simulink library "SEWSYS_library"  (Simulink 6.0)
settings: Solver=ode45  SolverMode=SingleTasking  StartTime=0.0  StopTime=10.0  RelTol=1e-3
values from neighbouring files (symbols this model uses):
  sec_per_ts = in_sec_per_ts    [Prep.m]
undefined symbols (not defined in the file or in its folder): DiscIntNeverNeededParam
settings Model: LastModifiedBy=v94ahlst
settings OptimizationCC: BooleanDataType=off
settings DebuggingCC: SolverPrmCheckMsg=none
settings HardwareCC: TargetUnknown=on

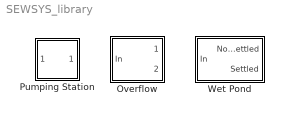
== system SEWSYS_library ==
  Overflow : Subsystem  mask(Overflow){choice=off, limit=0}
      mask prompts: choice "Overflow active"; limit "Overflow limit [m3/s]"
      mask help: Models an overflow
      mask Help:
      | To model an overflow:
      | First make the overflow active by the checkbox. Then enter the Overflow limit, ie the discharge threshold for which the overflow starts diverting. The signal from the first outport contains the bypassed part, the second outport the transit part.
  Pumping Station : Subsystem  mask(Pump){qp=, Ap=, ystart=, ynod=, ts=sec_per_ts}
      mask prompts: qp "Pump Capacity [m³/s]"; Ap "Pumping Pit Area [m²]"; ystart "Start Level [m] (Stop Level is ±0 m)"; ynod "Emergency Overflow Level [m]"; ts "Seconds per Timestep (DO NOT CHANGE THIS!)"
      mask help: Models a pumping station.
      mask Help: Enter the parameters
      mask Display: plot([0 1 5 6], [0 0 4 4])
  Wet Pond : Subsystem  mask(Wet Pond){Ap=0, d=0, n=1, vs=1.4977e-004, q_threshold=0.02, ts=sec_per_ts}
      mask prompts: Ap "Pond Area [m2]"; d "Average pond depth [m]"; n "Turbulence constant, n=1 poor performance (variable inflow)"; vs "Average settling velocity [m/s]"; q_threshold "Limit for dynamic settling [m3/s]"; ts "Seconds per Timestep (DO NOT CHANGE THIS!)"
      mask init:
      | partboundSS=[ ;% uncertain values, calculated from measurements (Pettersson et al, 1999 p.870)
      |    0.57      ;% P-tot
      |    0.10      ;% Tot-N
      |    0         ;% NH3/NH4-N
      |    0         ;% NO3-N
      |    0         ;% N2O-N
      |    0         ;% SS
      |    0.57      ;% BOD
      |    0         ;% COD
      |    0         ;% C-tot
      |    0         ;% Phase index
      |    0.43      ;% Cu
      |    0.43      ;% Zn
      |    0.71      ;% Pb
      |    0.16      ;% Cd
      |    0         ;% Hg
      |    0         ;% Cr
      |    0.90	    ;% Pt assumed values
      |    0.90	    ;% Pd ---"---
      |    0.90		 ;% Rh ---"---
      |    0.85      ;% PAH
      |    ]';

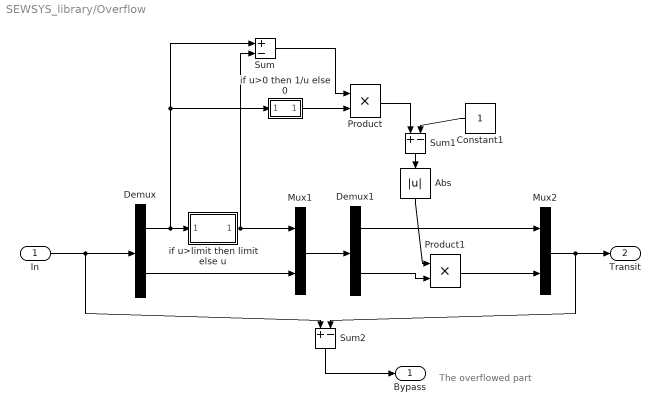
== system SEWSYS_library/Overflow ==
  note: The overflowed part
  In : Inport  Port=1  LatchInput=off
  Abs : Abs  Orientation=down  SaturateOnIntegerOverflow=on
  Constant1 : Constant  Orientation=left
  Demux : Demux  Outputs=[1 -1]
  Demux1 : Demux  Outputs=[1 -1]
  Mux1 : Mux  Inputs=2
  Mux2 : Mux  Inputs=2
  Product : Product  SaturateOnIntegerOverflow=on  InputSameDT=on
  Product1 : Product  SaturateOnIntegerOverflow=on  InputSameDT=on
  Sum : Sum  Inputs=+-  SaturateOnIntegerOverflow=on  InputSameDT=on
  Sum1 : Sum  Orientation=down  Inputs=+-  SaturateOnIntegerOverflow=on  InputSameDT=on
  Sum2 : Sum  Orientation=down  Inputs=+-  SaturateOnIntegerOverflow=on  InputSameDT=on
  if u>0 then 1/u else 0 : Subsystem
      mask Display: disp('1/u')
  if u>limit then limit else u : Subsystem
      mask Display: disp('Overflow')
  Bypass : Outport
  Transit : Outport  Port=2
  wires:
  Demux/2 -> Mux1/2
  Mux1/1 -> Demux1/1
  Demux1/1 -> Mux2/1
  Demux1/2 -> Product1/2
  Product1/1 -> Mux2/2
  if u>limit then limit else u/1(out_1) -> Sum/2, Mux1/1
  Constant1/1 -> Sum1/2
  Demux/1 -> if u>limit then limit else u/1(in_1), Sum/1, if u>0 then 1/u else 0/1(in_1)
  Sum1/1 -> Abs/1
  if u>0 then 1/u else 0/1(out_1) -> Product/2
  Sum2/1 -> Bypass/1
  In/1 -> Demux/1, Sum2/1
  Mux2/1 -> Transit/1, Sum2/2
  Product/1 -> Sum1/1
  Abs/1 -> Product1/1
  Sum/1 -> Product/1

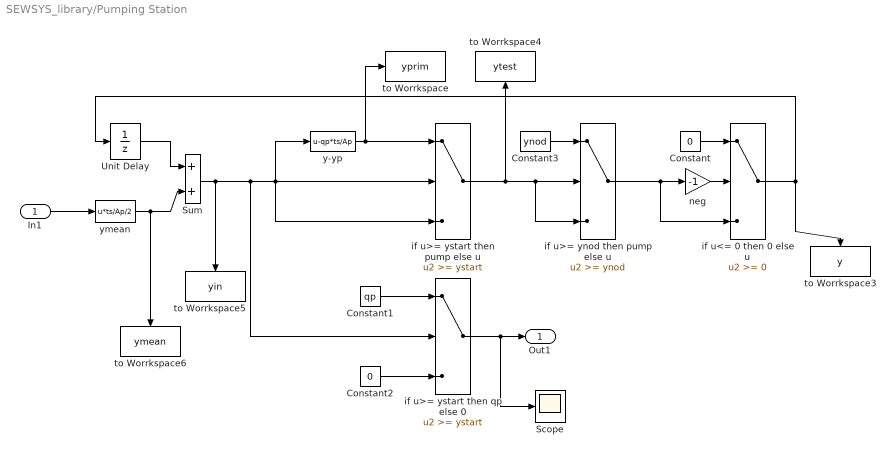
== system SEWSYS_library/Pumping Station ==
  In1 : Inport  Port=1  LatchInput=off
  Constant : Constant  Value=0
  Constant1 : Constant  Value=qp
  Constant2 : Constant  Value=0
  Constant3 : Constant  Value=ynod
  Scope : Scope
  Sum : Sum  SaturateOnIntegerOverflow=on  InputSameDT=on
  Unit Delay : UnitDelay
  if u<= 0 then 0 else u : Switch  SaturateOnIntegerOverflow=on  InputSameDT=on
  if u>= ynod then pump else u : Switch  Threshold=ynod  SaturateOnIntegerOverflow=on  InputSameDT=on
  if u>= ystart then pump else u : Switch  Threshold=ystart  SaturateOnIntegerOverflow=on  InputSameDT=on
  if u>= ystart then qp else 0 : Switch  Threshold=ystart  SaturateOnIntegerOverflow=on  InputSameDT=on
  neg : Gain  Gain=-1  SaturateOnIntegerOverflow=on
  to Worrkspace : ToWorkspace  VariableName=yprim  SampleTime=-1  SaveFormat=Array
  to Worrkspace3 : ToWorkspace  VariableName=y  SampleTime=-1  SaveFormat=Array
      settings: Orientation=down
  to Worrkspace4 : ToWorkspace  VariableName=ytest  SampleTime=-1  SaveFormat=Array
      settings: Orientation=up
  to Worrkspace5 : ToWorkspace  VariableName=yin  SampleTime=-1  SaveFormat=Array
      settings: Orientation=down
  to Worrkspace6 : ToWorkspace  VariableName=ymean  SampleTime=-1  SaveFormat=Array
      settings: Orientation=down
  y-yp : Fcn  Expr=u-qp*ts/Ap
  ymean : Fcn  Expr=u*ts/Ap/2
  Out1 : Outport
  wires:
  In1/1 -> ymean/1
  if u>= ystart then qp else 0/1 -> Scope/1, Out1/1
  Constant3/1 -> if u>= ynod then pump else u/1
  if u>= ystart then pump else u/1 -> if u>= ynod then pump else u/3, if u>= ynod then pump else u/2, to Worrkspace4/1
  if u>= ynod then pump else u/1 -> if u<= 0 then 0 else u/3, neg/1
  if u<= 0 then 0 else u/1 -> to Worrkspace3/1, Unit Delay/1
  neg/1 -> if u<= 0 then 0 else u/2
  Constant/1 -> if u<= 0 then 0 else u/1
  ymean/1 -> to Worrkspace6/1, Sum/2
  Constant2/1 -> if u>= ystart then qp else 0/3
  Constant1/1 -> if u>= ystart then qp else 0/1
  Sum/1 -> if u>= ystart then qp else 0/2, y-yp/1, if u>= ystart then pump else u/3, if u>= ystart then pump else u/2, to Worrkspace5/1
  y-yp/1 -> to Worrkspace/1, if u>= ystart then pump else u/1
  Unit Delay/1 -> Sum/1

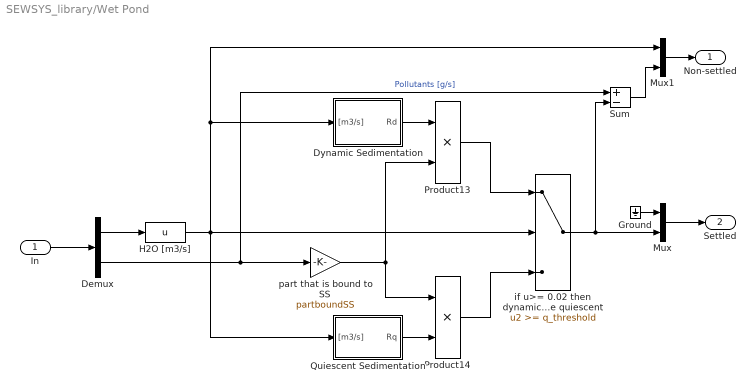
== system SEWSYS_library/Wet Pond ==
  In : Inport  Port=1  LatchInput=off
  Demux : Demux  Outputs=[1 -1]
  Dynamic Sedimentation : Subsystem
  Ground : Ground
  H2O [m3/s] : Fcn  Expr=u
  Mux : Mux  Inputs=2
  Mux1 : Mux  Inputs=2
  Product13 : Product  SaturateOnIntegerOverflow=on  InputSameDT=on
  Product14 : Product  SaturateOnIntegerOverflow=on  InputSameDT=on
  Quiescent Sedimentation : Subsystem
  Sum : Sum  Inputs=+-  SaturateOnIntegerOverflow=on  InputSameDT=on
  if u>= 0.02 then dynamic else quiescent : Switch  Threshold=q_threshold  SaturateOnIntegerOverflow=on  InputSameDT=on
  part that is bound to SS : Gain  Gain=partboundSS  SaturateOnIntegerOverflow=on
  Non-settled : Outport
  Settled : Outport  Port=2
  wires:
  part that is bound to SS/1 -> Product13/2, Product14/1
  Demux/2 -> part that is bound to SS/1, Sum/1  "Pollutants [g/s]"
  Mux1/1 -> Non-settled/1
  Sum/1 -> Mux1/2
  if u>= 0.02 then dynamic else quiescent/1 -> Sum/2, Mux/2
  Ground/1 -> Mux/1
  Mux/1 -> Settled/1
  Product14/1 -> if u>= 0.02 then dynamic else quiescent/3
  Product13/1 -> if u>= 0.02 then dynamic else quiescent/1
  Quiescent Sedimentation/1(Rq) -> Product14/2
  Dynamic Sedimentation/1(Rd) -> Product13/1
  In/1 -> Demux/1
  Demux/1 -> H2O [m3/s]/1
  H2O [m3/s]/1 -> Mux1/1, Dynamic Sedimentation/1("[m3/s]"), Quiescent Sedimentation/1("[m3/s]"), if u>= 0.02 then dynamic else quiescent/2

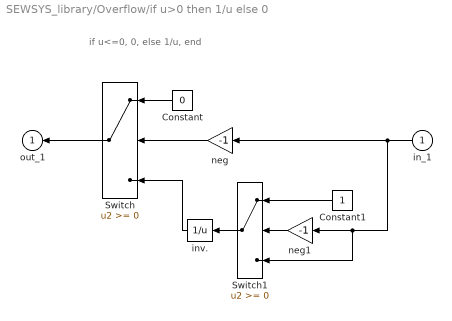
== system SEWSYS_library/Overflow/if u>0 then 1/u else 0 ==
  note: if u<=0, 0, else 1/u, end
  in_1 : Inport  Orientation=left  Port=1  LatchInput=off
  Constant : Constant  Orientation=left  Value=0
  Constant1 : Constant  Orientation=left
  Switch : Switch  Orientation=left  SaturateOnIntegerOverflow=on  InputSameDT=on
  Switch1 : Switch  Orientation=left  SaturateOnIntegerOverflow=on  InputSameDT=on
  inv. : Fcn  Orientation=left  Expr=1/u
  neg : Gain  Orientation=left  Gain=-1  SaturateOnIntegerOverflow=on
  neg1 : Gain  Orientation=left  Gain=-1  SaturateOnIntegerOverflow=on
  out_1 : Outport  Orientation=left  InitialOutput=0
  wires:
  Constant/1 -> Switch/1
  neg/1 -> Switch/2
  Switch/1 -> out_1/1
  inv./1 -> Switch/3
  Switch1/1 -> inv./1
  neg1/1 -> Switch1/2
  Constant1/1 -> Switch1/1
  in_1/1 -> neg/1, neg1/1, Switch1/3

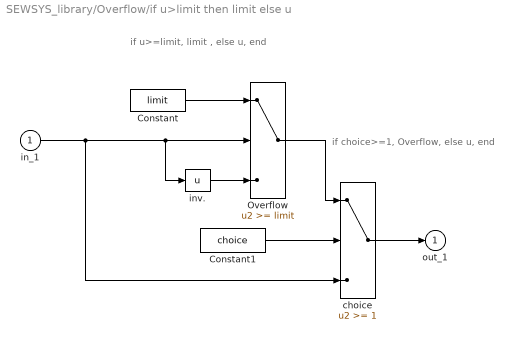
== system SEWSYS_library/Overflow/if u>limit then limit else u ==
  note: if u>=limit, limit
      | , else u, end
  note: if choice>=1, Overflow, else u, end
  in_1 : Inport  Port=1  LatchInput=off
  Constant : Constant  Value=limit
  Constant1 : Constant  Value=choice
  Overflow : Switch  Threshold=limit  SaturateOnIntegerOverflow=on  InputSameDT=on
  choice : Switch  Threshold=1  SaturateOnIntegerOverflow=on  InputSameDT=on
  inv. : Fcn  Expr=u
  out_1 : Outport  InitialOutput=0
  wires:
  Constant1/1 -> choice/2
  Constant/1 -> Overflow/1
  inv./1 -> Overflow/3
  Overflow/1 -> choice/1
  in_1/1 -> Overflow/2, inv./1, choice/3
  choice/1 -> out_1/1

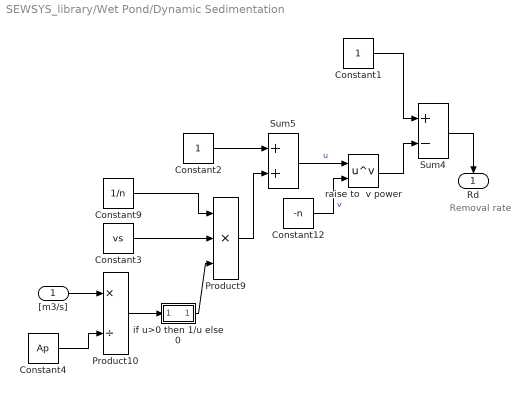
== system SEWSYS_library/Wet Pond/Dynamic Sedimentation ==
  note: Removal rate
  "[m3/s]" : Inport  Port=1  LatchInput=off
  Constant1 : Constant
  Constant12 : Constant  Value=-n
  Constant2 : Constant
  Constant3 : Constant  Value=vs
  Constant4 : Constant  Value=Ap
  Constant9 : Constant  Value=1/n
  Product10 : Product  Inputs=*/  SaturateOnIntegerOverflow=on  InputSameDT=on
  Product9 : Product  Inputs=3  SaturateOnIntegerOverflow=on  InputSameDT=on
  Sum4 : Sum  Inputs=+-  SaturateOnIntegerOverflow=on  InputSameDT=on
  Sum5 : Sum  SaturateOnIntegerOverflow=on  InputSameDT=on
  if u>0 then 1/u else 0 : Subsystem
      mask Display: disp('1/u')
  raise to  v power : Math  Operator=pow  SaturateOnIntegerOverflow=on
  Rd : Outport  Orientation=down
  wires:
  "[m3/s]"/1 -> Product10/1
  Constant4/1 -> Product10/2
  Product10/1 -> if u>0 then 1/u else 0/1(in_1)
  if u>0 then 1/u else 0/1(out_1) -> Product9/3
  Constant12/1 -> raise to  v power/2  "v"
  Constant9/1 -> Product9/1
  Constant3/1 -> Product9/2
  Product9/1 -> Sum5/2
  Constant2/1 -> Sum5/1
  Sum5/1 -> raise to  v power/1  "u"
  raise to  v power/1 -> Sum4/2
  Sum4/1 -> Rd/1
  Constant1/1 -> Sum4/1

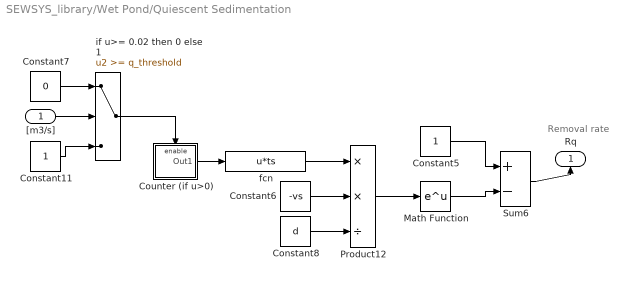
== system SEWSYS_library/Wet Pond/Quiescent Sedimentation ==
  note: Removal rate
  "[m3/s]" : Inport  Port=1  LatchInput=off
  Constant11 : Constant
  Constant5 : Constant
  Constant6 : Constant  Value=-vs
  Constant7 : Constant  Value=0
  Constant8 : Constant  Value=d
  Counter (if u>0) : Subsystem  TreatAsAtomicUnit=on
  Math Function : Math  SaturateOnIntegerOverflow=on
  Product12 : Product  Inputs=**/  SaturateOnIntegerOverflow=on  InputSameDT=on
  Sum6 : Sum  Inputs=+-  SaturateOnIntegerOverflow=on  InputSameDT=on
  fcn : Fcn  Expr=u*ts
  if u>= 0.02 then 0 else 1 : Switch  Threshold=q_threshold  SaturateOnIntegerOverflow=on  InputSameDT=on
  Rq : Outport  Orientation=up
  wires:
  Counter (if u>0)/1(Out1) -> fcn/1
  "[m3/s]"/1 -> if u>= 0.02 then 0 else 1/2
  if u>= 0.02 then 0 else 1/1 -> Counter (if u>0)/Enable
  Constant7/1 -> if u>= 0.02 then 0 else 1/1
  Constant11/1 -> if u>= 0.02 then 0 else 1/3
  fcn/1 -> Product12/1
  Constant8/1 -> Product12/3
  Constant6/1 -> Product12/2
  Product12/1 -> Math Function/1
  Constant5/1 -> Sum6/1
  Sum6/1 -> Rq/1
  Math Function/1 -> Sum6/2

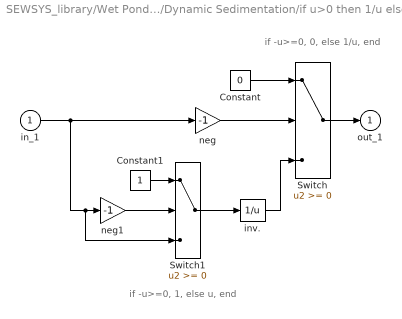
== system SEWSYS_library/Wet Pond/Dynamic Sedimentation/if u>0 then 1/u else 0 ==
  note: if -u>=0, 0, else 1/u, end
  note: if -u>=0, 1, else u, end
  in_1 : Inport  Port=1  LatchInput=off
  Constant : Constant  Value=0
  Constant1 : Constant
  Switch : Switch  SaturateOnIntegerOverflow=on  InputSameDT=on
  Switch1 : Switch  SaturateOnIntegerOverflow=on  InputSameDT=on
  inv. : Fcn  Expr=1/u
  neg : Gain  Gain=-1  SaturateOnIntegerOverflow=on
  neg1 : Gain  Gain=-1  SaturateOnIntegerOverflow=on
  out_1 : Outport  InitialOutput=0
  wires:
  Constant/1 -> Switch/1
  neg/1 -> Switch/2
  Switch/1 -> out_1/1
  inv./1 -> Switch/3
  Switch1/1 -> inv./1
  Constant1/1 -> Switch1/1
  neg1/1 -> Switch1/2
  in_1/1 -> neg/1, neg1/1, Switch1/3

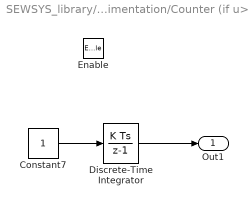
== system SEWSYS_library/Wet Pond/Quiescent Sedimentation/Counter (if u>0) ==
  Enable : EnablePort  StatesWhenEnabling=reset
  Constant7 : Constant
  Discrete-Time Integrator : DiscreteIntegrator  InitialCondition=1  ICPrevOutput=DiscIntNeverNeededParam  ICPrevScaledInput=DiscIntNeverNeededParam
  Out1 : Outport  InitialOutput=0
  wires:
  Discrete-Time Integrator/1 -> Out1/1
  Constant7/1 -> Discrete-Time Integrator/1
